simulink model "Microgrid_24h_Simulation"  (Simulink 9.3)
settings: Solver=ode45  StartTime=0.0  StopTime=1  RelTol=1e-3  EnableMultiTasking=on
undefined symbols (not defined in the file or in its folder): Acid, Lead
libraries: powerlib x60, powerlib_extras x56, simulink x3, powerlib_meascontrol x2, electricdrivelib x1
(part 1 of 3)
settings Model: Creator=Student  LastModifiedBy=DELL
settings DataIOCC: LimitDataPoints=on
settings OptimizationCC: ExpressionDepthLimit=2147483647
settings DebuggingCC: SolverPrmCheckMsg=warning  StateNameClashWarn=warning
settings GRTTargetCC: GeneratePreprocessorConditionals=Disable all
settings SimscapeCC: SimscapeNormalizeSystem=off

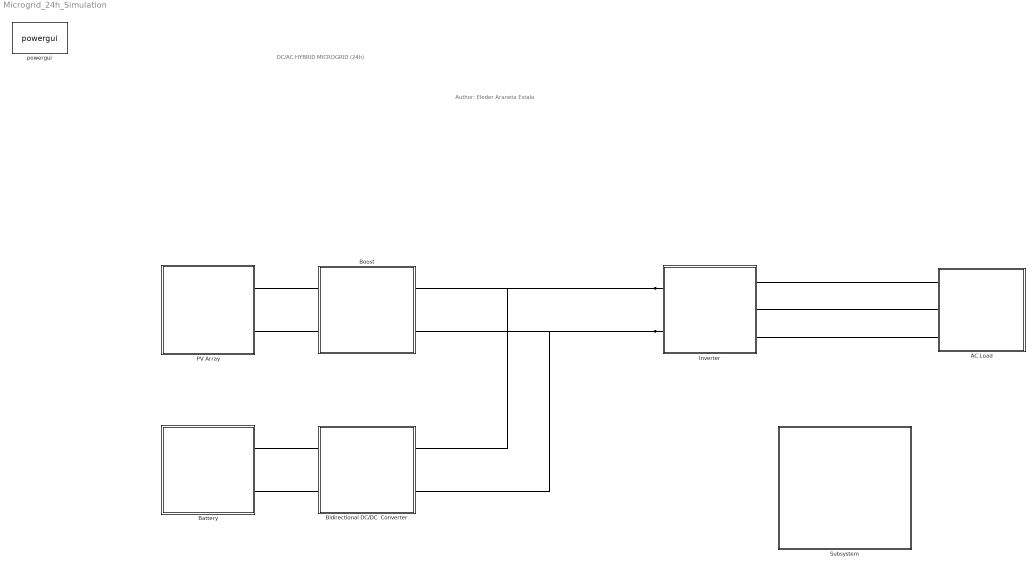
== system Microgrid_24h_Simulation ==
  note: DC/AC HYBRID MICROGRID (24h)
  note: Author: Eleder Araneta Estala
  AC Load : Subsystem
      mask Display: image(imread('Plug.bmp'))
  Battery : Subsystem
      mask Display: image(imread('Battery.bmp'))
  Bidirectional DC/DC  Converter : Subsystem
      mask Display: disp('Bidirectional Converter')
  Boost : Subsystem
      mask Display: disp('Boost Converter')
  Inverter : Subsystem
      mask Display: disp('DC/AC Inverter')
  PV Array : Subsystem
      mask Display: image(imread('photo.bmp'))
  Subsystem : Subsystem
      mask Display: disp('Measurements')
  powergui : powerlib/powergui  Priority=1  SimulationMode=Discrete  SampleTime=5e-6  frequency=60  Iterations=50  frequencyindice=0  Pbase=100e6  ErrMax=1e-4  UnitsV=kV  UnitsW=MW  buscounter=0  FunctionMessages=off  echomessages=off  EnableUseOfTLC=off  CurrentSourceSwitches=off  DisableSnubberDevices=off  DisableRonSwitches=off  DisableVfSwitches=off  DisplayEquations=off  AutomaticDiscreteSolvers=off  SolverType=Tustin  Interpol=off  ExternalGateDelay=off  methode=off  Ts=0  x0status=blocks  SPID=off  SwTol=0  HookPort=off  NonlinearTolerance=0  nMaxIteration=15  ContinueOnMaxIteration=off  RestoreLinks=warning  ResistiveCurrentMeasurement=off  Frange=[0:2:500]  Ylog=off  Xlog=on  ShowGrid=off  save=off  variable=ZData  structure=Vab_st  ZoomFFT=off  StartTime=7.5  cycles=4  DisplayStyle=1  fundamental=50  FreqAxis=off  MaxFrequency=50000  frequencyindicesteady=1  RmsSteady=1  display=off
      settings: SourceProductName=Simscape Electrical
  connections:
  Battery/LConn1 -- Bidirectional DC/DC  Converter/LConn1
  Battery/LConn2 -- Bidirectional DC/DC  Converter/LConn2
  PV Array/RConn2 -- Boost/LConn2
  PV Array/RConn1 -- Boost/LConn1
  Inverter/RConn1 -- Boost/RConn1 -- Bidirectional DC/DC  Converter/RConn1
  Inverter/RConn2 -- Boost/RConn2 -- Bidirectional DC/DC  Converter/RConn2
  AC Load/LConn3 -- Inverter/LConn3
  AC Load/LConn2 -- Inverter/LConn2
  AC Load/LConn1 -- Inverter/LConn1

== system Microgrid_24h_Simulation/AC Load ==
  3-Phase Dynamic Load : powerlib/Elements/Three-Phase Dynamic Load  NominalVoltage=[ 400 50 ]  ActiveReactivePowers=[25000 -500]  PositiveSequence=[1 0]  ExternalControl=off  NpNq="[1  1]"  TimeConstants="[0  0  0  0]"  MinimumVoltage=0.7  Tfilter=1e-4  LoadFlowParameters=[4 50000000 0 0 25000000]
      settings: SourceProductName=Simscape Electrical  SourceProductBaseCode=PS
  Bus Selector1 : BusSelector  OutputSignals=Active power P (W),Reactive power Q (var)  OutputAsBus=on
  Load Measurements : Subsystem
  Load Measurements1 : Subsystem
  Load Measurements2 : Scope
  Three-Phase Parallel RLC Load1 : powerlib/Elements/Three-Phase Parallel RLC Load  LConnTagsString=A|B|C  Configuration=Y (grounded)  NominalVoltage=400  Vabc=[1e3 1e3 1e3]  Vabcp=[1e3 1e3 1e3]  NominalFrequency=50  UnbalancedPower=off  ActivePower=700e3  InductivePower=0  CapacitivePower=0  Pabc=[10e3 9e3 11e3]  QLabc=[100 90 110]  QCabc=[100 90 110]  Pabcp=[10e3 9e3 11e3]  QLabcp=[100 90 110]  QCabcp=[100 90 110]  Measurements=Branch voltages and currents  LoadType=constant Z
      settings: SourceProductName=Simscape Electrical
  A : PMIOPort  Side=Left
  B : PMIOPort  Port=2  Side=Left
  C : PMIOPort  Port=3  Side=Left
  wires:
  3-Phase Dynamic Load/1 -> Bus Selector1/1
  Bus Selector1/1 -> Load Measurements2/1
  connections:
  A/RConn1 -- Load Measurements/LConn1 -- Load Measurements1/LConn1
  Load Measurements/LConn2 -- B/RConn1 -- Load Measurements1/LConn2
  Load Measurements/LConn3 -- C/RConn1 -- Load Measurements1/LConn3
  Load Measurements1/RConn1 -- Three-Phase Parallel RLC Load1/LConn1
  Load Measurements1/RConn2 -- Three-Phase Parallel RLC Load1/LConn2
  Load Measurements1/RConn3 -- Three-Phase Parallel RLC Load1/LConn3
  Load Measurements/RConn1 -- 3-Phase Dynamic Load/LConn1
  Load Measurements/RConn2 -- 3-Phase Dynamic Load/LConn2
  Load Measurements/RConn3 -- 3-Phase Dynamic Load/LConn3

== system Microgrid_24h_Simulation/Battery ==
  Battery : electricdrivelib/Extra Sources/Battery  BatType=Lead-Acid  ShowTempParam=off  ThermalPreset=no  ShowAgeParam=off  NomV=250  NomQ=500  SOC=30  Batt_Tr=1  PresetModel=on  MaxQ=520.8333  MinV=187.5  FullV=272.2039  Dis_rate=100  R=0.005  Normal_OP=155.1389  expZone="[254.523      1.666667]"  current=[20 50 100]  Units=Time  Tci=20  NomT=20  T2=-30  MaxQ2=4.8  FullV2=7.1  Normal_OP2=5.655  expZone2="[6.58           1]"  Rca=0.6  ti=2000  Dp=0  Neq0=0  Tsim=1e6  Ta1=25  Qeol=5.4*0.9  Reol=0.013333*1.2  Char_age=[2.3478, 3]  Dis_age=[2.3478, 10]  N1=1500  N2=10500  N3=1000  N4=1400  Ta2=45  N5=950
      settings: SourceProductName=Simscape Electrical
  Bus Selector : BusSelector  OutputSignals=SOC (%),Current (A),Voltage (V)
  LPF vq1 : powerlib_extras/Discrete  Control Blocks/Discrete 1st-Order Filter  FilterType=Lowpass  Tc=10e-3  Ts=5e-6  Initialize=off  Vac_Init=[0.8 -25 60]  Vdc_Init=0  PlotResponse=off  param1=[1 100 0.1]
      settings: SourceProductName=Simscape Electrical  SourceProductBaseCode=PS
  LPF vq2 : powerlib_extras/Discrete  Control Blocks/Discrete 1st-Order Filter  FilterType=Lowpass  Tc=10e-3  Ts=5e-6  Initialize=off  Vac_Init=[0.8 -25 60]  Vdc_Init=0  PlotResponse=off  param1=[1 100 0.1]
      settings: SourceProductName=Simscape Electrical  SourceProductBaseCode=PS
  Subsystem1 : Subsystem
  Subsystem2 : Subsystem
  Subsystem5 : Subsystem
  + : PMIOPort  Side=Left
  - : PMIOPort  Port=2  Side=Left
  wires:
  Battery/1 -> Bus Selector/1
  Bus Selector/2 -> LPF vq1/1  "<Current (A)>"
  LPF vq1/1 -> Subsystem1/1(Ibat)
  Bus Selector/1 -> Subsystem5/1(SOC)  "<SOC (%)>"
  Bus Selector/3 -> LPF vq2/1  "<Voltage (V)>"
  LPF vq2/1 -> Subsystem2/1(Vbat)
  connections:
  -/RConn1 -- Battery/LConn2
  Battery/LConn1 -- +/RConn1

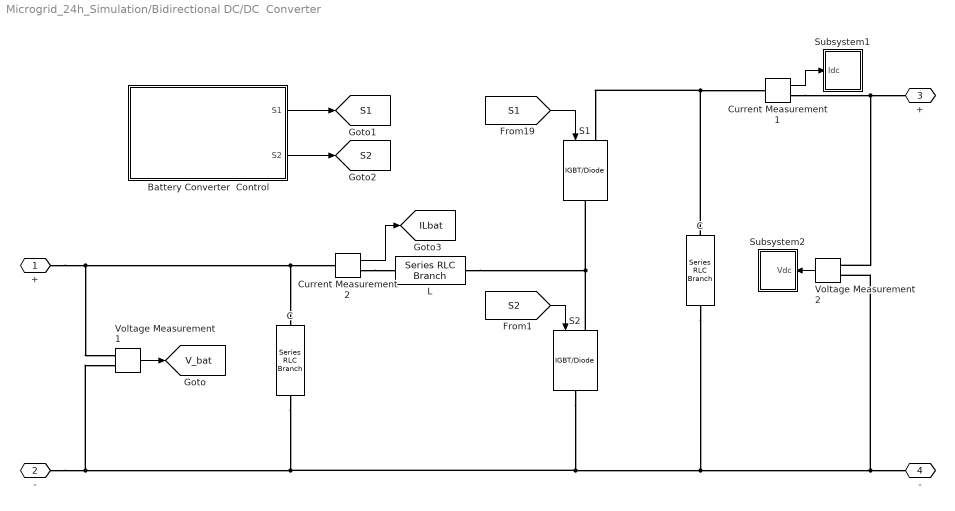
== system Microgrid_24h_Simulation/Bidirectional DC/DC  Converter ==
  Battery Converter  Control : Subsystem
  C : powerlib/Elements/Series RLC Branch  LConnTagsString=__new0  RConnTagsString=__new0  BranchType=C  Resistance=1  Inductance=1e-3  SetiL0=off  InitialCurrent=0  Capacitance=1200e-6  Setx0=off  InitialVoltage=400  Measurements=None
      settings: SourceProductName=Simscape Electrical
  "C " : powerlib/Elements/Series RLC Branch  LConnTagsString=__new0  RConnTagsString=__new0  BranchType=C  Resistance=1  Inductance=1e-3  SetiL0=off  InitialCurrent=0  Capacitance=1e-3  Setx0=on  InitialVoltage=192  Measurements=None
      settings: SourceProductName=Simscape Electrical
  Current Measurement1 : powerlib/Measurements/Current Measurement  PhasorSimulation=off  OutputType=Complex  PSBequivalent=0
      settings: SourceProductName=Simscape Electrical
  Current Measurement2 : powerlib/Measurements/Current Measurement  PhasorSimulation=off  OutputType=Complex  PSBequivalent=0
      settings: SourceProductName=Simscape Electrical
  L : powerlib/Elements/Series RLC Branch  LConnTagsString=__new0  RConnTagsString=__new0  BranchType=L  Resistance=1  Inductance=0.1e-3  SetiL0=on  InitialCurrent=0  Capacitance=1e-6  Setx0=off  InitialVoltage=0  Measurements=None
      settings: SourceProductName=Simscape Electrical
  "S1 " : powerlib/Power Electronics/IGBT//Diode  Ron=1e-3  Rs=1e5  Cs=inf  Measurements=off
      settings: SourceProductName=Simscape Electrical
  "S2 " : powerlib/Power Electronics/IGBT//Diode  Ron=1e-3  Rs=1e5  Cs=inf  Measurements=off
      settings: SourceProductName=Simscape Electrical
  Subsystem1 : Subsystem
  Subsystem2 : Subsystem
  Voltage Measurement1 : powerlib/Measurements/Voltage Measurement  PhasorSimulation=off  OutputType=Complex  PSBequivalent=0
      settings: SourceProductName=Simscape Electrical
  Voltage Measurement2 : powerlib/Measurements/Voltage Measurement  PhasorSimulation=off  OutputType=Complex  PSBequivalent=0
      settings: SourceProductName=Simscape Electrical
  "+ " : PMIOPort  Side=Left
  "-  " : PMIOPort  Port=2  Side=Left
  + : PMIOPort  Port=3  Side=Right
  - : PMIOPort  Port=4  Side=Right
  tag scope: ILbat=global, S1=global, S2=global, V_bat=global
  wires:
  Voltage Measurement1/1 -> [V_bat]
  Current Measurement2/1 -> [ILbat]
  Battery Converter  Control/1(S1) -> [S1]
  Battery Converter  Control/2(S2) -> [S2]
  [S1] -> "S1 "/1
  [S2] -> "S2 "/1
  Voltage Measurement2/1 -> Subsystem2/1(Vdc)
  Current Measurement1/1 -> Subsystem1/1(Idc)
  connections:
  "-  "/RConn1 -- Voltage Measurement1/LConn2 -- "C "/RConn1 -- "S2 "/RConn1 -- C/RConn1 -- -/RConn1 -- Voltage Measurement2/LConn2
  "S2 "/LConn1 -- "S1 "/RConn1 -- L/RConn1
  C/LConn1 -- "S1 "/LConn1 -- Current Measurement1/LConn1
  Current Measurement2/RConn1 -- L/LConn1
  "+ "/RConn1 -- Voltage Measurement1/LConn1 -- Current Measurement2/LConn1 -- "C "/LConn1
  Current Measurement1/RConn1 -- +/RConn1 -- Voltage Measurement2/LConn1

== system Microgrid_24h_Simulation/Boost ==
  Cdc : powerlib/Elements/Series RLC Branch  LConnTagsString=__new0  RConnTagsString=__new0  BranchType=C  Resistance=1  Inductance=1e-3  SetiL0=off  InitialCurrent=0  Capacitance=1200e-6  Setx0=off  InitialVoltage=400  Measurements=None
      settings: SourceProductName=Simscape Electrical
  Current Measurement : powerlib/Measurements/Current Measurement  PhasorSimulation=off  OutputType=Complex  PSBequivalent=0
      settings: SourceProductName=Simscape Electrical
  Current Measurement1 : powerlib/Measurements/Current Measurement  PhasorSimulation=off  OutputType=Complex  PSBequivalent=0
      settings: SourceProductName=Simscape Electrical
  Diode : powerlib/Power Electronics/Diode  Ron=0.001  Lon=0  Vf=0.8  IC=0  UseSnubber=off  Rs=500  Cs=250e-9  Measurements=on
      settings: SourceProductName=Simscape Electrical
  IGBT/Diode : powerlib/Power Electronics/IGBT//Diode  Ron=1e-3  Rs=1e5  Cs=inf  Measurements=off
      settings: SourceProductName=Simscape Electrical
  Incremental Conductance MPPT : Subsystem
  Lb : powerlib/Elements/Series RLC Branch  LConnTagsString=__new0  RConnTagsString=__new0  BranchType=L  Resistance=1  Inductance=880e-6  SetiL0=off  InitialCurrent=0  Capacitance=1e-6  Setx0=off  InitialVoltage=0  Measurements=None
      settings: SourceProductName=Simscape Electrical
  Subsystem1 : Subsystem
  Subsystem2 : Subsystem
  Va : powerlib/Measurements/Voltage Measurement  PhasorSimulation=off  OutputType=Complex  PSBequivalent=0
      settings: SourceProductName=Simscape Electrical
  Voltage Measurement : powerlib/Measurements/Voltage Measurement  PhasorSimulation=off  OutputType=Complex  PSBequivalent=0
      settings: SourceProductName=Simscape Electrical
  + : PMIOPort  Side=Left
  - : PMIOPort  Port=2  Side=Left
  "+ " : PMIOPort  Port=3  Side=Right
  "- " : PMIOPort  Port=4  Side=Right
  tag scope: IL=global, S=global, Vin=global
  wires:
  Current Measurement/1 -> [IL]
  [S] -> IGBT/Diode/1
  Voltage Measurement/1 -> Subsystem2/1(Vbus)
  Current Measurement1/1 -> Subsystem1/1(Ibus)
  Va/1 -> [Vin]
  Incremental Conductance MPPT/1(Pulsos) -> [S]
  connections:
  Voltage Measurement/LConn1 -- Current Measurement1/LConn1 -- Diode/RConn1 -- Cdc/LConn1
  Cdc/RConn1 -- "- "/RConn1 -- Voltage Measurement/LConn2 -- -/RConn1 -- Va/LConn2 -- IGBT/Diode/RConn1
  Lb/RConn1 -- Current Measurement/LConn1
  IGBT/Diode/LConn1 -- Current Measurement/RConn1 -- Diode/LConn1
  +/RConn1 -- Lb/LConn1 -- Va/LConn1
  "+ "/RConn1 -- Current Measurement1/RConn1

== system Microgrid_24h_Simulation/Inverter ==
  DC / AC Inverter : Subsystem
  "DC BUS " : Subsystem
  Inverter Control : Subsystem
  Inverter Control1 : Subsystem
  + : PMIOPort  Side=Right
  A : PMIOPort  Port=2  Side=Left
  B : PMIOPort  Port=3  Side=Left
  - : PMIOPort  Port=4  Side=Right
  C : PMIOPort  Port=5  Side=Left
  wires:
  Inverter Control/1(S) -> DC / AC Inverter/1(S)
  connections:
  A/RConn1 -- DC / AC Inverter/LConn1
  B/RConn1 -- DC / AC Inverter/LConn2
  C/RConn1 -- DC / AC Inverter/LConn3
  "DC BUS "/LConn2 -- DC / AC Inverter/RConn2
  "DC BUS "/LConn1 -- DC / AC Inverter/RConn1
  +/RConn1 -- "DC BUS "/RConn1
  -/RConn1 -- "DC BUS "/RConn2

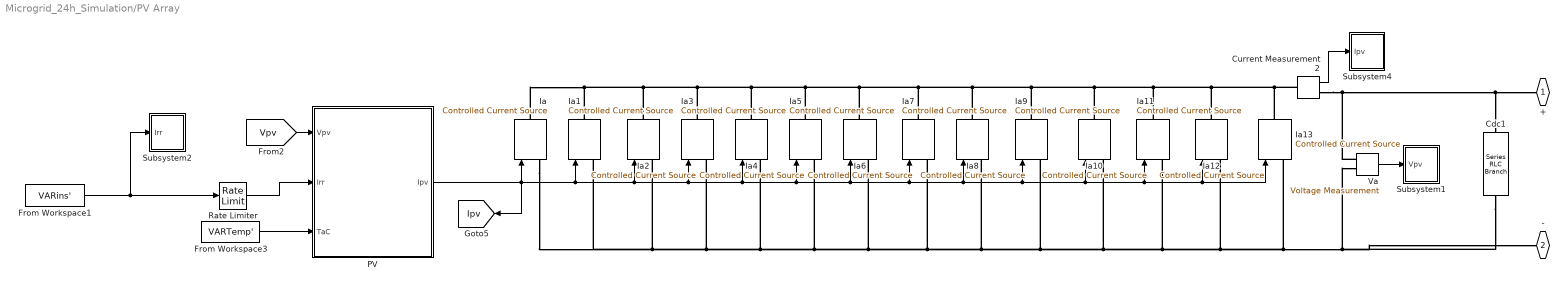
== system Microgrid_24h_Simulation/PV Array ==
  Cdc1 : powerlib/Elements/Series RLC Branch  LConnTagsString=__new0  RConnTagsString=__new0  BranchType=C  Resistance=1  Inductance=1e-3  SetiL0=off  InitialCurrent=0  Capacitance=5e-3  Setx0=off  InitialVoltage=192  Measurements=None
      settings: SourceProductName=Simscape Electrical
  Current Measurement2 : powerlib/Measurements/Current Measurement  PhasorSimulation=off  OutputType=Complex  PSBequivalent=0
      settings: SourceProductName=Simscape Electrical
  From Workspace1 : FromWorkspace  VariableName=VARins'  SampleTime=0
  From Workspace3 : FromWorkspace  VariableName=VARTemp'  SampleTime=0
  Ia{,1..13} (14 alike) : powerlib/Electrical Sources/Controlled Current Source  Initialize=on  Source_Type=DC  Amplitude=0  Phase=0  Frequency=0  Measurements=None
      settings: SourceProductName=Simscape Electrical
  PV : MATLAB Function  TreatAsAtomicUnit=on
  Rate Limiter : RateLimiter  RisingSlewLimit=5  FallingSlewLimit=-5
  Subsystem1 : Subsystem
  Subsystem2 : Subsystem
  Subsystem4 : Subsystem
  Va : powerlib/Measurements/Voltage Measurement  PhasorSimulation=off  OutputType=Complex  PSBequivalent=0
      settings: SourceProductName=Simscape Electrical
  + : PMIOPort  Side=Right
  - : PMIOPort  Port=2  Side=Right
  tag scope: Ipv=global
  wires:
  [Vpv] -> PV/1(Vpv)
  PV/1(Ipv) -> Ia/1, [Ipv], Ia1/1, Ia2/1, Ia3/1, Ia4/1, Ia5/1, Ia6/1, Ia7/1, Ia8/1, Ia9/1, Ia10/1, Ia11/1, Ia13/1, Ia12/1
  Va/1 -> Subsystem1/1(Vpv)
  Rate Limiter/1 -> PV/2(Irr)
  Current Measurement2/1 -> Subsystem4/1(Ipv)
  From Workspace3/1 -> PV/3(TaC)
  From Workspace1/1 -> Subsystem2/1(Irr), Rate Limiter/1
  connections:
  Ia/LConn1 -- Ia1/LConn1 -- Ia2/LConn1 -- Ia3/LConn1 -- Ia4/LConn1 -- Ia5/LConn1 -- Ia6/LConn1 -- Ia7/LConn1 -- Ia8/LConn1 -- Ia9/LConn1 -- Ia10/LConn1 -- Ia11/LConn1 -- Ia12/LConn1 -- Va/LConn2 -- Cdc1/RConn1 -- -/RConn1 -- Ia13/LConn1
  Current Measurement2/LConn1 -- Ia/RConn1 -- Ia1/RConn1 -- Ia2/RConn1 -- Ia3/RConn1 -- Ia4/RConn1 -- Ia5/RConn1 -- Ia6/RConn1 -- Ia7/RConn1 -- Ia8/RConn1 -- Ia9/RConn1 -- Ia10/RConn1 -- Ia11/RConn1 -- Ia12/RConn1 -- Ia13/RConn1
  Va/LConn1 -- Current Measurement2/RConn1 -- +/RConn1 -- Cdc1/LConn1

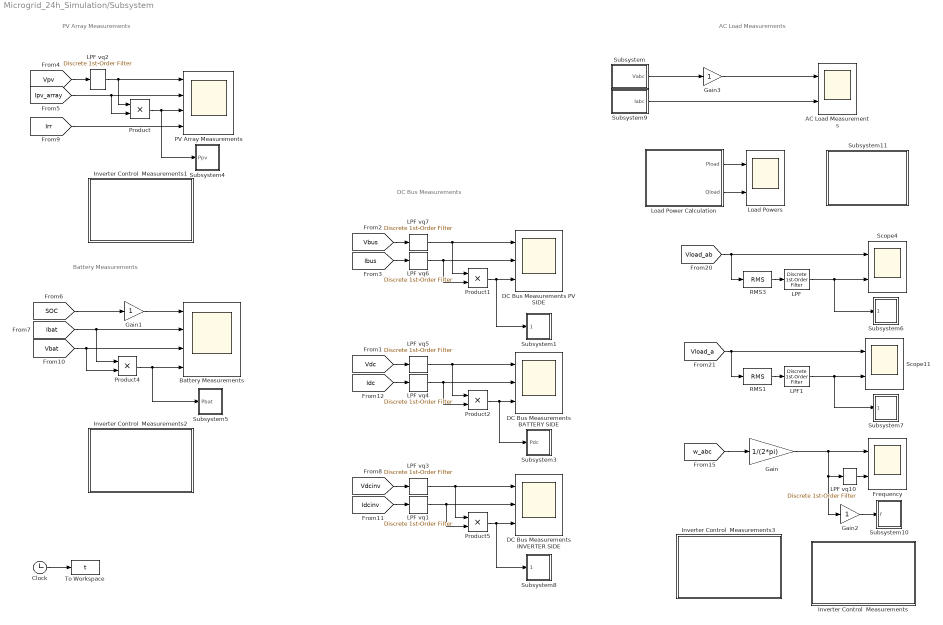
== system Microgrid_24h_Simulation/Subsystem ==
  note: PV Array Measurements
  note: Battery Measurements
  note: DC Bus Measurements
  note: AC Load Measurements
  AC Load Measurements : Scope  NumInputPorts=2
  Battery Measurements : Scope  NumInputPorts=4
  Clock : Clock
  DC Bus Measurements BATTERY SIDE : Scope  NumInputPorts=3
  DC Bus Measurements INVERTER SIDE : Scope  NumInputPorts=3
  DC Bus Measurements PV SIDE : Scope  NumInputPorts=3
  Frequency : Scope  NumInputPorts=2
  Gain : Gain  Gain=1/(2*pi)
  Gain1 : Gain
  Gain2 : Gain
  Gain3 : Gain
  Inverter Control  Measurements : Subsystem
      mask Display: disp('Inverter Control')
  Inverter Control  Measurements1 : Subsystem
      mask Display: disp('Boost Converter Control')
  Inverter Control  Measurements2 : Subsystem
      mask Display: disp('Bidirectional Converter Control')
  Inverter Control  Measurements3 : Subsystem
      mask Display: disp('Frequency Measurement')
  LPF : powerlib_extras/Discrete  Control Blocks/Discrete 1st-Order Filter  FilterType=Lowpass  Tc=10e-3  Ts=5e-6  Initialize=off  Vac_Init=[0.8 -25 60]  Vdc_Init=0  PlotResponse=off  param1=[1 100 0.1]
      settings: SourceProductName=Simscape Electrical  SourceProductBaseCode=PS
  LPF vq{1..7,10} (8 alike) : powerlib_extras/Discrete  Control Blocks/Discrete 1st-Order Filter  FilterType=Lowpass  Tc=10e-3  Ts=5e-6  Initialize=off  Vac_Init=[0.8 -25 60]  Vdc_Init=0  PlotResponse=off  param1=[1 100 0.1]
      settings: SourceProductName=Simscape Electrical  SourceProductBaseCode=PS
  LPF1 : powerlib_extras/Discrete  Control Blocks/Discrete 1st-Order Filter  FilterType=Lowpass  Tc=10e-3  Ts=5e-6  Initialize=off  Vac_Init=[0.8 -25 60]  Vdc_Init=0  PlotResponse=off  param1=[1 100 0.1]
      settings: SourceProductName=Simscape Electrical  SourceProductBaseCode=PS
  Load Power Calculation : Subsystem
  Load Powers : Scope  NumInputPorts=2
  PV Array Measurements : Scope  NumInputPorts=4
  Product{,1..2,4..5} (5 alike) : Product  RndMeth=Zero
  RMS1 : powerlib_extras/Measurements/RMS  f1=60
      settings: SourceProductName=Simscape Electrical  SourceProductBaseCode=PS
  RMS3 : powerlib_extras/Measurements/RMS  f1=60
      settings: SourceProductName=Simscape Electrical  SourceProductBaseCode=PS
  Scope11 : Scope  NumInputPorts=2
  Scope4 : Scope  NumInputPorts=2
  Subsystem : Subsystem
  Subsystem1 : Subsystem
  Subsystem10 : Subsystem
  Subsystem11 : Subsystem
      mask Display: disp('Additional Load Meas.')
  Subsystem3 : Subsystem
  Subsystem4 : Subsystem
  Subsystem5 : Subsystem
  Subsystem6 : Subsystem
  Subsystem7 : Subsystem
  Subsystem8 : Subsystem
  Subsystem9 : Subsystem
  To Workspace : ToWorkspace  VariableName=t  SampleTime=5e-6
  wires:
  Product/1 -> PV Array Measurements/3, Subsystem4/1(Ppv)
  [Vpv] -> LPF vq2/1
  [Ipv_array] -> PV Array Measurements/2, Product/2
  [Irr] -> PV Array Measurements/4
  [SOC] -> Gain1/1
  [Ibat] -> Battery Measurements/2, Product4/1
  [Vbat] -> Battery Measurements/3, Product4/2
  Product4/1 -> Battery Measurements/4, Subsystem5/1(Pbat)
  [Vdc] -> LPF vq5/1
  [Idc] -> LPF vq4/1
  Product2/1 -> DC Bus Measurements BATTERY SIDE/3, Subsystem3/1(Pdc)
  Product1/1 -> DC Bus Measurements PV SIDE/3, Subsystem1/1(Pbus)
  [Vbus] -> LPF vq7/1
  [Ibus] -> LPF vq6/1
  Load Power Calculation/1(Pload) -> Load Powers/1
  Load Power Calculation/2(Qload) -> Load Powers/2
  [Vload_a] -> Scope11/1, RMS1/1
  RMS1/1 -> LPF1/1
  [Vload_ab] -> Scope4/1, RMS3/1
  RMS3/1 -> LPF/1
  LPF/1 -> Scope4/2, Subsystem6/1(Vab_rms)
  LPF1/1 -> Scope11/2, Subsystem7/1(Va_rms)
  Clock/1 -> To Workspace/1
  Product5/1 -> Subsystem8/1(Pdcinv), DC Bus Measurements INVERTER SIDE/3
  [Vdcinv] -> LPF vq3/1
  [Idcinv] -> LPF vq1/1
  LPF vq2/1 -> PV Array Measurements/1, Product/1
  LPF vq1/1 -> DC Bus Measurements INVERTER SIDE/2, Product5/2
  LPF vq3/1 -> DC Bus Measurements INVERTER SIDE/1, Product5/1
  LPF vq4/1 -> Product2/2, DC Bus Measurements BATTERY SIDE/2
  LPF vq5/1 -> Product2/1, DC Bus Measurements BATTERY SIDE/1
  LPF vq6/1 -> DC Bus Measurements PV SIDE/2, Product1/2
  LPF vq7/1 -> DC Bus Measurements PV SIDE/1, Product1/1
  [w_abc] -> Gain/1
  Gain/1 -> Frequency/1, LPF vq10/1, Gain2/1
  LPF vq10/1 -> Frequency/2
  Subsystem9/1(Iabc) -> AC Load Measurements/2
  Subsystem/1(Vabc) -> Gain3/1
  Gain1/1 -> Battery Measurements/1
  Gain2/1 -> Subsystem10/1(f)
  Gain3/1 -> AC Load Measurements/1

== system Microgrid_24h_Simulation/AC Load/Load Measurements ==
  Subsystem1 : Subsystem
  Subsystem2 : Subsystem
  Three-Phase V Measurement : powerlib/Measurements/Three-Phase V-I Measurement  VoltageMeasurement=phase-to-ground  SetLabelV=off  LabelV=Vabc  Vpu=off  VpuLL=off  CurrentMeasurement=no  SetLabelI=off  LabelI=Iabc  Ipu=off  Pbase=100e6  Vbase=500e3  OutputType=Complex  PhasorSimulation=off  PSBequivalent=0
      settings: SourceProductName=Simscape Electrical
  Three-Phase  I Measurement : powerlib/Measurements/Three-Phase V-I Measurement  VoltageMeasurement=no  SetLabelV=off  LabelV=Vabc  Vpu=off  VpuLL=off  CurrentMeasurement=yes  SetLabelI=off  LabelI=Iabc  Ipu=off  Pbase=100e6  Vbase=500e3  OutputType=Complex  PhasorSimulation=off  PSBequivalent=0
      settings: SourceProductName=Simscape Electrical
  A : PMIOPort  Side=Left
  "A " : PMIOPort  Port=2  Side=Right
  B : PMIOPort  Port=3  Side=Left
  "B " : PMIOPort  Port=4  Side=Right
  C : PMIOPort  Port=5  Side=Left
  "C " : PMIOPort  Port=6  Side=Right
  wires:
  Three-Phase  I Measurement/1 -> Subsystem2/1(Iabc)
  Three-Phase V Measurement/1 -> Subsystem1/1(Vabc)
  connections:
  Three-Phase V Measurement/LConn1 -- Three-Phase  I Measurement/RConn1
  Three-Phase V Measurement/LConn2 -- Three-Phase  I Measurement/RConn2
  Three-Phase  I Measurement/RConn3 -- Three-Phase V Measurement/LConn3
  A/RConn1 -- Three-Phase  I Measurement/LConn1
  Three-Phase V Measurement/RConn1 -- "A "/RConn1
  B/RConn1 -- Three-Phase  I Measurement/LConn2
  Three-Phase V Measurement/RConn2 -- "B "/RConn1
  C/RConn1 -- Three-Phase  I Measurement/LConn3
  Three-Phase V Measurement/RConn3 -- "C "/RConn1

== system Microgrid_24h_Simulation/AC Load/Load Measurements1 ==
  Subsystem1 : Subsystem
  Subsystem2 : Subsystem
  Three-Phase V Measurement : powerlib/Measurements/Three-Phase V-I Measurement  VoltageMeasurement=phase-to-ground  SetLabelV=off  LabelV=Vabc  Vpu=off  VpuLL=off  CurrentMeasurement=no  SetLabelI=off  LabelI=Iabc  Ipu=off  Pbase=100e6  Vbase=500e3  OutputType=Complex  PhasorSimulation=off  PSBequivalent=0
      settings: SourceProductName=Simscape Electrical
  Three-Phase  I Measurement : powerlib/Measurements/Three-Phase V-I Measurement  VoltageMeasurement=no  SetLabelV=off  LabelV=Vabc  Vpu=off  VpuLL=off  CurrentMeasurement=yes  SetLabelI=off  LabelI=Iabc  Ipu=off  Pbase=100e6  Vbase=500e3  OutputType=Complex  PhasorSimulation=off  PSBequivalent=0
      settings: SourceProductName=Simscape Electrical
  a : PMIOPort  Side=Left
  "A " : PMIOPort  Port=2  Side=Right
  B : PMIOPort  Port=3  Side=Left
  "B " : PMIOPort  Port=4  Side=Right
  C : PMIOPort  Port=5  Side=Left
  "C " : PMIOPort  Port=6  Side=Right
  wires:
  Three-Phase V Measurement/1 -> Subsystem1/1(Vabc)
  Three-Phase  I Measurement/1 -> Subsystem2/1(Iabc3)
  connections:
  Three-Phase V Measurement/RConn3 -- "C "/RConn1
  C/RConn1 -- Three-Phase  I Measurement/LConn3
  Three-Phase V Measurement/RConn2 -- "B "/RConn1
  B/RConn1 -- Three-Phase  I Measurement/LConn2
  Three-Phase V Measurement/RConn1 -- "A "/RConn1
  a/RConn1 -- Three-Phase  I Measurement/LConn1
  Three-Phase  I Measurement/RConn3 -- Three-Phase V Measurement/LConn3
  Three-Phase V Measurement/LConn2 -- Three-Phase  I Measurement/RConn2
  Three-Phase V Measurement/LConn1 -- Three-Phase  I Measurement/RConn1

== system Microgrid_24h_Simulation/Battery/Subsystem1 ==
  Ibat : Inport
  To Workspace1 : ToWorkspace  VariableName=Ibat  SampleTime=-1
  tag scope: Ibat=global
  wires:
  Ibat/1 -> To Workspace1/1, [Ibat]

== system Microgrid_24h_Simulation/Battery/Subsystem2 ==
  Vbat : Inport
  To Workspace1 : ToWorkspace  VariableName=Vbat  SampleTime=-1
  tag scope: Vbat=global
  wires:
  Vbat/1 -> To Workspace1/1, [Vbat]

== system Microgrid_24h_Simulation/Battery/Subsystem5 ==
  SOC : Inport
  To Workspace1 : ToWorkspace  VariableName=SOC  SampleTime=-1
  tag scope: SOC=global
  wires:
  SOC/1 -> To Workspace1/1, [SOC]

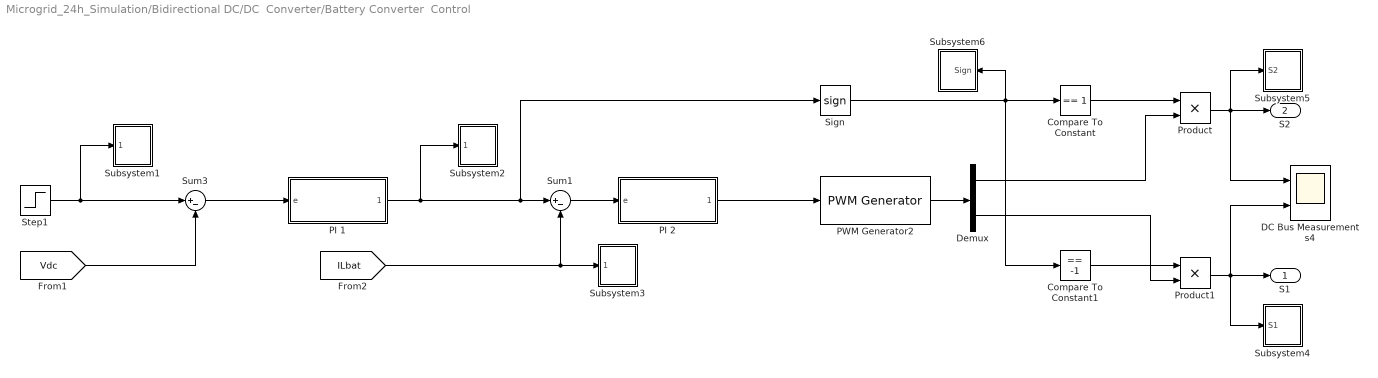
== system Microgrid_24h_Simulation/Bidirectional DC/DC  Converter/Battery Converter  Control ==
  Compare To Constant : simulink/Logic and Bit Operations/Compare To Constant  relop===  const=1  OutDataTypeStr=uint8
  Compare To Constant1 : simulink/Logic and Bit Operations/Compare To Constant  relop===  const=-1  OutDataTypeStr=uint8
  DC Bus Measurements4 : Scope  NumInputPorts=2
  Demux : Demux  Outputs=2
  PI 1 : Subsystem
  PI 2 : Subsystem
  PWM Generator2 : powerlib_extras/Control  Blocks/PWM Generator  GeneratorMode="1-arm  bridge (2 pulses)"  Fc=10000  Internal=off  mIndex=0.2  Freq=0  Phase=0
      link override Triangle: rep_seq_y=[0 1 0]  rep_seq_t=[0 1/Fc/2 1/Fc]
      settings: SourceProductName=Simscape Electrical  SourceProductBaseCode=PS
  Product : Product  RndMeth=Zero
  Product1 : Product  RndMeth=Zero
  Sign : Signum  SampleTime=5e-6
  Step1 : Step  Time=0  After=1000  SampleTime=0
  Subsystem1 : Subsystem
  Subsystem2 : Subsystem
  Subsystem3 : Subsystem
  Subsystem4 : Subsystem
  Subsystem5 : Subsystem
  Subsystem6 : Subsystem
  Sum1 : Sum  Inputs=|+-
  Sum3 : Sum  Inputs=|+-
  S1 : Outport
  S2 : Outport  Port=2
  wires:
  Step1/1 -> Sum3/1, Subsystem1/1(Vdc_ref)
  Sum3/1 -> PI 1/1(e)
  Sum1/1 -> PI 2/1(e)
  [ILbat] -> Sum1/2, Subsystem3/1(ILbat)
  PI 1/1(" ") -> Sum1/1, Sign/1, Subsystem2/1(Ibat_ref)
  PI 2/1(" ") -> PWM Generator2/1
  PWM Generator2/1 -> Demux/1
  Sign/1 -> Compare To Constant/1, Compare To Constant1/1, Subsystem6/1(Sign)
  Compare To Constant/1 -> Product/1
  Demux/1 -> Product/2
  Compare To Constant1/1 -> Product1/1
  Product/1 -> DC Bus Measurements4/1, S2/1, Subsystem5/1(S2)
  Product1/1 -> S1/1, Subsystem4/1(S1), DC Bus Measurements4/2
  Demux/2 -> Product1/2
  [Vdc] -> Sum3/2

== system Microgrid_24h_Simulation/Bidirectional DC/DC  Converter/Subsystem1 ==
  Idc : Inport
  LPF vq11 : powerlib_extras/Discrete  Control Blocks/Discrete 1st-Order Filter  FilterType=Lowpass  Tc=10e-3  Ts=5e-6  Initialize=off  Vac_Init=[0.8 -25 60]  Vdc_Init=0  PlotResponse=off  param1=[1 100 0.1]
      settings: SourceProductName=Simscape Electrical  SourceProductBaseCode=PS
  To Workspace1 : ToWorkspace  VariableName=Idc  SampleTime=-1
  To Workspace2 : ToWorkspace  VariableName=Idc1  SampleTime=-1
  tag scope: Idc=global
  wires:
  Idc/1 -> [Idc], To Workspace1/1, LPF vq11/1
  LPF vq11/1 -> To Workspace2/1

== system Microgrid_24h_Simulation/Bidirectional DC/DC  Converter/Subsystem2 ==
  Vdc : Inport
  LPF vq11 : powerlib_extras/Discrete  Control Blocks/Discrete 1st-Order Filter  FilterType=Lowpass  Tc=10e-3  Ts=5e-6  Initialize=off  Vac_Init=[0.8 -25 60]  Vdc_Init=0  PlotResponse=off  param1=[1 100 0.1]
      settings: SourceProductName=Simscape Electrical  SourceProductBaseCode=PS
  To Workspace1 : ToWorkspace  VariableName=Vdc  SampleTime=-1
  To Workspace2 : ToWorkspace  VariableName=Vdc1  SampleTime=-1
  tag scope: Vdc=global
  wires:
  Vdc/1 -> [Vdc], To Workspace1/1, LPF vq11/1
  LPF vq11/1 -> To Workspace2/1

== system Microgrid_24h_Simulation/Boost/Incremental Conductance MPPT ==
  Demux : Demux  Outputs=2
  MPPT IC : MATLAB Function  TreatAsAtomicUnit=on
  Memory{,1..2,4..5} (5 alike) : Memory
  PWM Generator : powerlib_extras/Control  Blocks/PWM Generator  GeneratorMode="1-arm  bridge (2 pulses)"  Fc=10e3  Internal=off  mIndex=0.4  Freq=60  Phase=0
      link override Triangle: rep_seq_t=[0 1/Fc/2 1/Fc]  rep_seq_y=[0 1 0]
      settings: SourceProductName=Simscape Electrical  SourceProductBaseCode=PS
  Subsystem1 : Subsystem
  Subsystem2 : Subsystem
  Subsystem3 : Subsystem
  Pulsos : Outport
  wires:
  Memory2/1 -> MPPT IC/4(Vprevious)
  Memory5/1 -> MPPT IC/5(Vref_previous)
  Memory4/1 -> MPPT IC/2(Iprevious)
  Memory1/1 -> MPPT IC/3(Vpv)
  Memory/1 -> MPPT IC/1(Ipv)
  PWM Generator/1 -> Demux/1
  Demux/2 -> Pulsos/1, Subsystem3/1(pulsos)
  MPPT IC/1(delta) -> Subsystem2/1(delta), PWM Generator/1
  MPPT IC/3(Ipv_prev_out) -> Memory4/1
  MPPT IC/4(Vpv_prev_out) -> Memory2/1
  MPPT IC/2(Vref) -> Memory5/1, Subsystem1/1(Vref)
  [Ipv] -> Memory/1
  [Vpv] -> Memory1/1

== system Microgrid_24h_Simulation/Boost/Subsystem1 ==
  Ibus : Inport
  LPF vq11 : powerlib_extras/Discrete  Control Blocks/Discrete 1st-Order Filter  FilterType=Lowpass  Tc=10e-3  Ts=5e-6  Initialize=off  Vac_Init=[0.8 -25 60]  Vdc_Init=0  PlotResponse=off  param1=[1 100 0.1]
      settings: SourceProductName=Simscape Electrical  SourceProductBaseCode=PS
  To Workspace1 : ToWorkspace  VariableName=Ibus  SampleTime=-1
  To Workspace2 : ToWorkspace  VariableName=Ibus1  SampleTime=-1
  tag scope: Ibus=global
  wires:
  Ibus/1 -> [Ibus], To Workspace1/1, LPF vq11/1
  LPF vq11/1 -> To Workspace2/1

== system Microgrid_24h_Simulation/Boost/Subsystem2 ==
  Vbus : Inport
  LPF vq11 : powerlib_extras/Discrete  Control Blocks/Discrete 1st-Order Filter  FilterType=Lowpass  Tc=10e-3  Ts=5e-6  Initialize=off  Vac_Init=[0.8 -25 60]  Vdc_Init=0  PlotResponse=off  param1=[1 100 0.1]
      settings: SourceProductName=Simscape Electrical  SourceProductBaseCode=PS
  To Workspace1 : ToWorkspace  VariableName=Vbus  SampleTime=-1
  To Workspace2 : ToWorkspace  VariableName=Vbus1  SampleTime=-1
  tag scope: Vbus=global
  wires:
  Vbus/1 -> [Vbus], To Workspace1/1, LPF vq11/1
  LPF vq11/1 -> To Workspace2/1

== system Microgrid_24h_Simulation/Inverter/DC / AC Inverter ==
  S : Inport
  2 Level Inverter : powerlib/Power Electronics/Universal Bridge  Arms=3  SnubberResistance=1e5  SnubberCapacitance=inf  Device=IGBT / Diodes  Ron=1e-3  Lon=0  ForwardVoltages="[  0  0  ]"  ForwardVoltage=0  GTOparameters=[ 10e-6 , 20e-6 ]  IGBTparameters=[ 1e-6 , 2e-6 ]  Measurements=UAB UBC UCA UDC voltages  Measurements_2=None  converterType=Rectifier
      settings: SourceProductName=Simscape Electrical
  AC Load Measurements : Subsystem
  Series RLC Branch1 : powerlib/Elements/Series RLC Branch  LConnTagsString=__new0  RConnTagsString=__new0  BranchType=RL  Resistance=0.1  Inductance=30e-3  SetiL0=off  InitialCurrent=0  Capacitance=1e-6  Setx0=off  InitialVoltage=0  Measurements=Branch voltage
      settings: SourceProductName=Simscape Electrical
  Series RLC Branch2 : powerlib/Elements/Series RLC Branch  LConnTagsString=__new0  RConnTagsString=__new0  BranchType=RL  Resistance=0.1  Inductance=30e-3  SetiL0=off  InitialCurrent=0  Capacitance=1e-6  Setx0=off  InitialVoltage=0  Measurements=Branch voltage
      settings: SourceProductName=Simscape Electrical
  Series RLC Branch3 : powerlib/Elements/Series RLC Branch  LConnTagsString=__new0  RConnTagsString=__new0  BranchType=RL  Resistance=0.1  Inductance=30e-3  SetiL0=off  InitialCurrent=0  Capacitance=1e-6  Setx0=off  InitialVoltage=0  Measurements=Branch voltage
      settings: SourceProductName=Simscape Electrical
  + : PMIOPort  Side=Right
  A : PMIOPort  Port=2  Side=Left
  B : PMIOPort  Port=3  Side=Left
  - : PMIOPort  Port=4  Side=Right
  C : PMIOPort  Port=5  Side=Left
  wires:
  S/1 -> 2 Level Inverter/1
  connections:
  2 Level Inverter/RConn1 -- +/RConn1
  2 Level Inverter/RConn2 -- -/RConn1
  Series RLC Branch2/LConn1 -- 2 Level Inverter/LConn1
  2 Level Inverter/LConn2 -- Series RLC Branch1/LConn1
  2 Level Inverter/LConn3 -- Series RLC Branch3/LConn1
  Series RLC Branch2/RConn1 -- AC Load Measurements/LConn1
  Series RLC Branch1/RConn1 -- AC Load Measurements/LConn2
  Series RLC Branch3/RConn1 -- AC Load Measurements/LConn3
  AC Load Measurements/RConn1 -- A/RConn1
  AC Load Measurements/RConn2 -- B/RConn1
  AC Load Measurements/RConn3 -- C/RConn1

== system Microgrid_24h_Simulation/Inverter/DC BUS  ==
  Current Measurement1 : powerlib/Measurements/Current Measurement  PhasorSimulation=off  OutputType=Complex  PSBequivalent=0
      settings: SourceProductName=Simscape Electrical
  DC Bus : powerlib/Elements/Series RLC Branch  LConnTagsString=__new0  RConnTagsString=__new0  BranchType=C  Resistance=1  Inductance=5e-03  SetiL0=off  InitialCurrent=0  Capacitance=10e-3/2  Setx0=off  InitialVoltage=1000/2  Measurements=None
      settings: SourceProductName=Simscape Electrical
  "DC Bus " : powerlib/Elements/Series RLC Branch  LConnTagsString=__new0  RConnTagsString=__new0  BranchType=C  Resistance=1  Inductance=5e-03  SetiL0=off  InitialCurrent=0  Capacitance=10e-3/2  Setx0=off  InitialVoltage=1000/2  Measurements=None
      settings: SourceProductName=Simscape Electrical
  Ground : powerlib/Elements/Ground  LConnTagsString=a
      settings: SourceProductName=Simscape Electrical
  Subsystem1 : Subsystem
  Subsystem2 : Subsystem
  Voltage Measurement1 : powerlib/Measurements/Voltage Measurement  PhasorSimulation=off  OutputType=Complex  PSBequivalent=0
      settings: SourceProductName=Simscape Electrical
  "+ " : PMIOPort  Side=Left
  "- " : PMIOPort  Port=2  Side=Left
  "+  " : PMIOPort  Port=3  Side=Right
  "-  " : PMIOPort  Port=4  Side=Right
  wires:
  Voltage Measurement1/1 -> Subsystem2/1(Vdcinv)
  Current Measurement1/1 -> Subsystem1/1(Idcinv)
  connections:
  DC Bus/LConn1 -- "+  "/RConn1 -- Voltage Measurement1/LConn1 -- Current Measurement1/LConn1
  "DC Bus "/LConn1 -- DC Bus/RConn1 -- Ground/LConn1
  "DC Bus "/RConn1 -- "-  "/RConn1 -- "- "/RConn1 -- Voltage Measurement1/LConn2
  Current Measurement1/RConn1 -- "+ "/RConn1

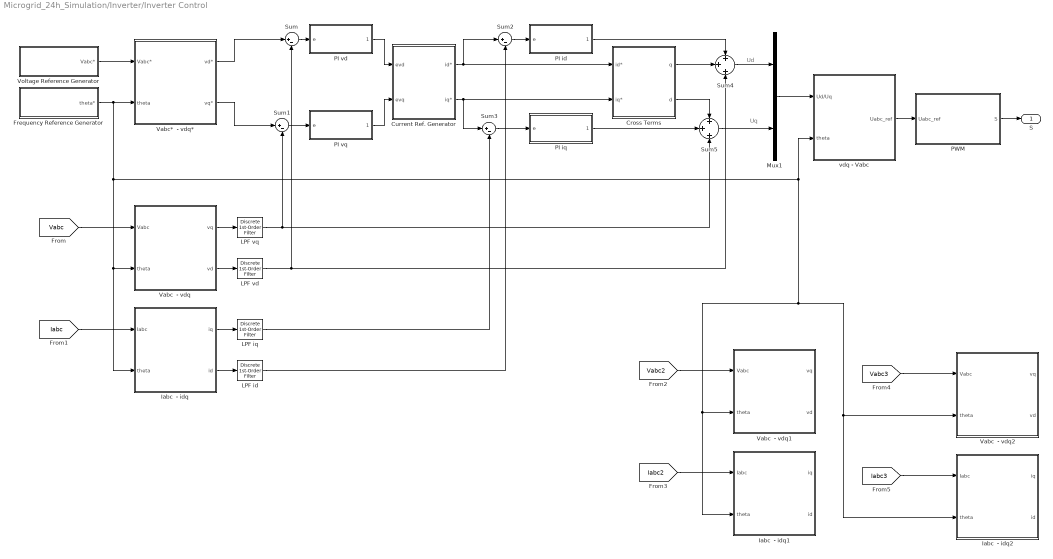
== system Microgrid_24h_Simulation/Inverter/Inverter Control ==
  note: Ud
  note: Uq
  " Voltage Reference Generator" : Subsystem
  Cross Terms : Subsystem
  Current Ref. Generator : Subsystem
  Frequency Reference Generator : Subsystem
  Iabc  - idq : Subsystem
  Iabc  - idq1 : Subsystem
  Iabc  - idq2 : Subsystem
  LPF id : powerlib_extras/Discrete  Control Blocks/Discrete 1st-Order Filter  FilterType=Lowpass  Tc=1e-3  Ts=5e-6  Initialize=off  Vac_Init=[0.8 -25 60]  Vdc_Init=0  PlotResponse=off  param1=[1 100 0.1]
      settings: SourceProductName=Simscape Electrical  SourceProductBaseCode=PS
  LPF iq : powerlib_extras/Discrete  Control Blocks/Discrete 1st-Order Filter  FilterType=Lowpass  Tc=1e-3  Ts=5e-6  Initialize=off  Vac_Init=[0.8 -25 60]  Vdc_Init=0  PlotResponse=off  param1=[1 100 0.1]
      settings: SourceProductName=Simscape Electrical  SourceProductBaseCode=PS
  LPF vd : powerlib_extras/Discrete  Control Blocks/Discrete 1st-Order Filter  FilterType=Lowpass  Tc=10e-3  Ts=5e-6  Initialize=off  Vac_Init=[0.8 -25 60]  Vdc_Init=-0.4  PlotResponse=off  param1=[1 100 0.1]
      settings: SourceProductName=Simscape Electrical  SourceProductBaseCode=PS
  LPF vq : powerlib_extras/Discrete  Control Blocks/Discrete 1st-Order Filter  FilterType=Lowpass  Tc=10e-3  Ts=5e-6  Initialize=off  Vac_Init=[0.8 -25 60]  Vdc_Init=0  PlotResponse=off  param1=[1 100 0.1]
      settings: SourceProductName=Simscape Electrical  SourceProductBaseCode=PS
  Mux1 : Mux  Inputs=2
  PI id : Subsystem
  PI iq : Subsystem
  PI vd : Subsystem
  PI vq : Subsystem
  PWM : Subsystem
  Sum{,1..3} (4 alike) : Sum  Inputs=|+-
  Sum4 : Sum  Inputs=+|+|+
  Sum5 : Sum  Inputs=+|+|+
  Vabc  - vdq : Subsystem
  Vabc  - vdq1 : Subsystem
  Vabc  - vdq2 : Subsystem
  Vabc*  - vdq* : Subsystem
  vdq - Vabc : Subsystem
  S : Outport
  wires:
  [Vabc] -> Vabc  - vdq/1(Vabc)
  [Iabc] -> Iabc  - idq/1(Iabc)
  Sum2/1 -> PI id/1(e)
  Sum3/1 -> PI iq/1(e)
  Mux1/1 -> vdq - Vabc/1(Ud/Uq)
  vdq - Vabc/1(Uabc_ref) -> PWM/1(Uabc_ref)
  PWM/1(S) -> S/1
  Vabc  - vdq/2(vd) -> LPF vd/1
  Iabc  - idq/1(iq) -> LPF iq/1
  Iabc  - idq/2(id) -> LPF id/1
  LPF vd/1 -> Sum/2, Sum4/3
  LPF vq/1 -> Sum1/2, Sum5/3
  LPF iq/1 -> Sum3/2
  LPF id/1 -> Sum2/2
  Sum/1 -> PI vd/1(e)
  Sum1/1 -> PI vq/1(e)
  Vabc  - vdq/1(vq) -> LPF vq/1
  Vabc*  - vdq*/1(vd*) -> Sum/1
  Vabc*  - vdq*/2(vq*) -> Sum1/1
  " Voltage Reference Generator"/1(Vabc*) -> Vabc*  - vdq*/1(Vabc*)
  Frequency Reference Generator/1(theta*) -> Vabc*  - vdq*/2(theta), Vabc  - vdq/2(theta), Iabc  - idq/2(theta), vdq - Vabc/2(theta), Vabc  - vdq2/2(theta), Iabc  - idq2/2(theta), Iabc  - idq1/2(theta), Vabc  - vdq1/2(theta)
  PI vd/1(" ") -> Current Ref. Generator/1(evd)
  PI vq/1(" ") -> Current Ref. Generator/2(evq)
  Current Ref. Generator/2(iq*) -> Sum3/1, Cross Terms/2(iq*)
  Current Ref. Generator/1(id*) -> Sum2/1, Cross Terms/1(id*)
  PI iq/1(" ") -> Sum5/2
  PI id/1(" ") -> Sum4/1
  Cross Terms/1(" q") -> Sum4/2
  Cross Terms/2(" d") -> Sum5/1
  Sum5/1 -> Mux1/2
  Sum4/1 -> Mux1/1
  [Vabc2] -> Vabc  - vdq1/1(Vabc)
  [Iabc2] -> Iabc  - idq1/1(Iabc)
  [Vabc3] -> Vabc  - vdq2/1(Vabc)
  [Iabc3] -> Iabc  - idq2/1(Iabc)

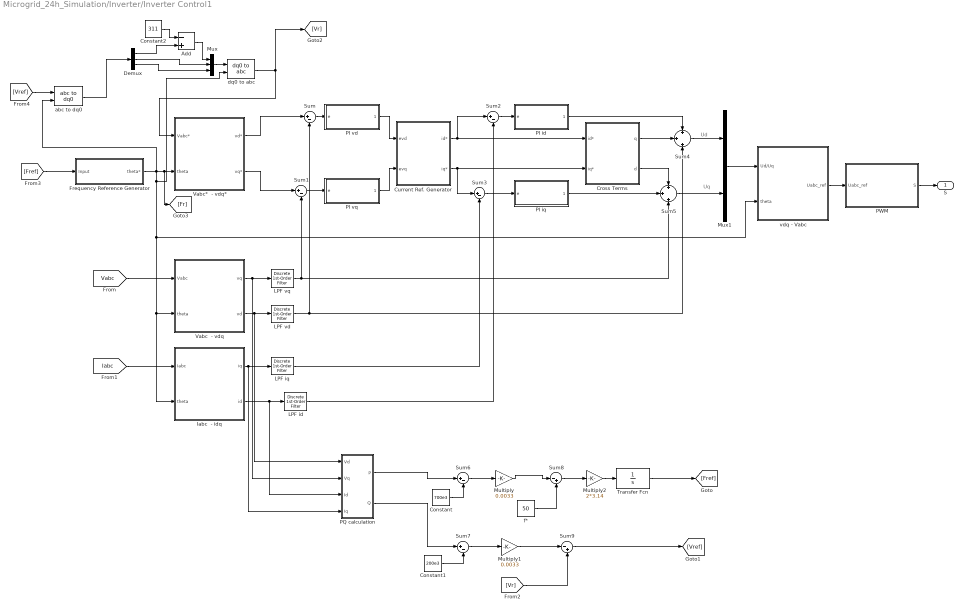
== system Microgrid_24h_Simulation/Inverter/Inverter Control1 ==
  note: Ud
  note: Uq
  Add : Sum  Inputs=-+
  Constant : Constant  Value=700e3
  Constant1 : Constant  Value=200e3
  Constant2 : Constant  Value=311
  Cross Terms : Subsystem
  Current Ref. Generator : Subsystem
  Demux : Demux  Outputs=3
  Frequency Reference Generator : Subsystem
  Iabc  - idq : Subsystem
  LPF id : powerlib_extras/Discrete  Control Blocks/Discrete 1st-Order Filter  FilterType=Lowpass  Tc=1e-3  Ts=5e-6  Initialize=off  Vac_Init=[0.8 -25 60]  Vdc_Init=0  PlotResponse=off  param1=[1 100 0.1]
      settings: SourceProductName=Simscape Electrical  SourceProductBaseCode=PS
  LPF iq : powerlib_extras/Discrete  Control Blocks/Discrete 1st-Order Filter  FilterType=Lowpass  Tc=1e-3  Ts=5e-6  Initialize=off  Vac_Init=[0.8 -25 60]  Vdc_Init=0  PlotResponse=off  param1=[1 100 0.1]
      settings: SourceProductName=Simscape Electrical  SourceProductBaseCode=PS
  LPF vd : powerlib_extras/Discrete  Control Blocks/Discrete 1st-Order Filter  FilterType=Lowpass  Tc=10e-3  Ts=5e-6  Initialize=off  Vac_Init=[0.8 -25 60]  Vdc_Init=-0.4  PlotResponse=off  param1=[1 100 0.1]
      settings: SourceProductName=Simscape Electrical  SourceProductBaseCode=PS
  LPF vq : powerlib_extras/Discrete  Control Blocks/Discrete 1st-Order Filter  FilterType=Lowpass  Tc=10e-3  Ts=5e-6  Initialize=off  Vac_Init=[0.8 -25 60]  Vdc_Init=0  PlotResponse=off  param1=[1 100 0.1]
      settings: SourceProductName=Simscape Electrical  SourceProductBaseCode=PS
  Multiply : Gain  Gain=0.0033
  Multiply1 : Gain  Gain=0.0033
  Multiply2 : Gain  Gain=2*3.14
  Mux : Mux  Inputs=3
  Mux1 : Mux  Inputs=2
  PI id : Subsystem
  PI iq : Subsystem
  PI vd : Subsystem
  PI vq : Subsystem
  PQ calculation : Subsystem
  PWM : Subsystem
  Sum{,1..3,6..7} (6 alike) : Sum  Inputs=|+-
  Sum4 : Sum  Inputs=+|+|+
  Sum5 : Sum  Inputs=+|+|+
  Sum8 : Sum  Inputs=|-+
  Sum9 : Sum  Inputs=|-+
  Transfer Fcn : TransferFcn  Denominator=[0 1 0]
  Vabc  - vdq : Subsystem
  Vabc*  - vdq* : Subsystem
  abc to dq0 : powerlib_meascontrol/Transformations/abc to dq0  Alignment=90 degrees behind phase A axis
      settings: SourceProductName=Simscape Electrical
  dq0 to abc : powerlib_meascontrol/Transformations/dq0 to abc  Alignment=90 degrees behind phase A axis
      settings: SourceProductName=Simscape Electrical
  "f* " : Constant  Value=50
  vdq - Vabc : Subsystem
  S : Outport
  wires:
  [Vabc] -> Vabc  - vdq/1(Vabc)
  [Iabc] -> Iabc  - idq/1(Iabc)
  Sum2/1 -> PI id/1(e)
  Sum3/1 -> PI iq/1(e)
  Mux1/1 -> vdq - Vabc/1(Ud/Uq)
  vdq - Vabc/1(Uabc_ref) -> PWM/1(Uabc_ref)
  PWM/1(S) -> S/1
  Vabc  - vdq/2(vd) -> PQ calculation/1(Vd), LPF vd/1
  Iabc  - idq/1(iq) -> PQ calculation/4(Iq), LPF iq/1
  Iabc  - idq/2(id) -> PQ calculation/3(Id), LPF id/1
  LPF vd/1 -> Sum/2, Sum4/3
  LPF vq/1 -> Sum1/2, Sum5/3
  LPF iq/1 -> Sum3/2
  LPF id/1 -> Sum2/2
  Sum/1 -> PI vd/1(e)
  Sum1/1 -> PI vq/1(e)
  Vabc  - vdq/1(vq) -> PQ calculation/2(Vq), LPF vq/1
  Vabc*  - vdq*/1(vd*) -> Sum/1
  Vabc*  - vdq*/2(vq*) -> Sum1/1
  dq0 to abc/1 -> [Vr], Vabc*  - vdq*/1(Vabc*)
  Frequency Reference Generator/1(theta*) -> dq0 to abc/2, Vabc  - vdq/2(theta), Iabc  - idq/2(theta), vdq - Vabc/2(theta), abc to dq0/2, [Fr], Vabc*  - vdq*/2(theta)
  PI vd/1(" ") -> Current Ref. Generator/1(evd)
  PI vq/1(" ") -> Current Ref. Generator/2(evq)
  Current Ref. Generator/2(iq*) -> Sum3/1, Cross Terms/2(iq*)
  Current Ref. Generator/1(id*) -> Sum2/1, Cross Terms/1(id*)
  PI iq/1(" ") -> Sum5/2
  PI id/1(" ") -> Sum4/1
  Cross Terms/1(" q") -> Sum4/2
  Cross Terms/2(" d") -> Sum5/1
  Sum5/1 -> Mux1/2
  Sum4/1 -> Mux1/1
  Constant1/1 -> Sum7/2
  Sum8/1 -> Multiply2/1
  Multiply/1 -> Sum8/1
  Multiply2/1 -> Transfer Fcn/1
  Constant/1 -> Sum6/2
  [Vr] -> Sum9/2
  "f* "/1 -> Sum8/2
  Sum7/1 -> Multiply1/1
  Multiply1/1 -> Sum9/1
  Sum6/1 -> Multiply/1
  PQ calculation/1(P) -> Sum6/1
  PQ calculation/2(Q) -> Sum7/1
  Transfer Fcn/1 -> [Fref]
  Sum9/1 -> [Vref]
  [Fref] -> Frequency Reference Generator/1(Input)
  [Vref] -> abc to dq0/1
  abc to dq0/1 -> Demux/1
  Constant2/1 -> Add/1
  Demux/1 -> Add/2
  Add/1 -> Mux/1
  Demux/2 -> Mux/2
  Demux/3 -> Mux/3
  Mux/1 -> dq0 to abc/1

== system Microgrid_24h_Simulation/PV Array/Subsystem1 ==
  Vpv : Inport
  LPF vq2 : powerlib_extras/Discrete  Control Blocks/Discrete 1st-Order Filter  FilterType=Lowpass  Tc=10e-3  Ts=5e-6  Initialize=off  Vac_Init=[0.8 -25 60]  Vdc_Init=0  PlotResponse=off  param1=[1 100 0.1]
      settings: SourceProductName=Simscape Electrical  SourceProductBaseCode=PS
  To Workspace1 : ToWorkspace  VariableName=Vpv  SampleTime=-1
  tag scope: Vpv=global
  wires:
  Vpv/1 -> [Vpv], LPF vq2/1
  LPF vq2/1 -> To Workspace1/1

== system Microgrid_24h_Simulation/PV Array/Subsystem2 ==
  Irr : Inport
  To Workspace1 : ToWorkspace  VariableName=Irr  SampleTime=-1
  Zero-Order Hold : ZeroOrderHold  SampleTime=5e-6
  tag scope: Irr=global
  wires:
  Irr/1 -> Zero-Order Hold/1
  Zero-Order Hold/1 -> To Workspace1/1, [Irr]

== system Microgrid_24h_Simulation/PV Array/Subsystem4 ==
  Ipv : Inport
  To Workspace1 : ToWorkspace  VariableName=Ipv_array  SampleTime=-1
  tag scope: Ipv_array=global
  wires:
  Ipv/1 -> [Ipv_array], To Workspace1/1

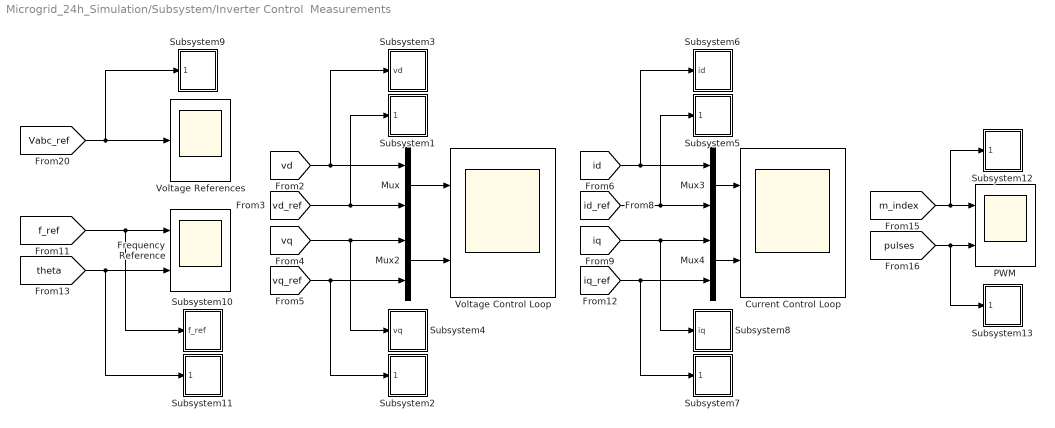
== system Microgrid_24h_Simulation/Subsystem/Inverter Control  Measurements ==
  Current Control Loop : Scope  NumInputPorts=2
  Frequency Reference : Scope  NumInputPorts=2
  Mux{,2..4} (4 alike) : Mux  Inputs=2
  PWM : Scope  NumInputPorts=2
  Subsystem1 : Subsystem
  Subsystem10 : Subsystem
  Subsystem11 : Subsystem
  Subsystem12 : Subsystem
  Subsystem13 : Subsystem
  Subsystem2 : Subsystem
  Subsystem3 : Subsystem
  Subsystem4 : Subsystem
  Subsystem5 : Subsystem
  Subsystem6 : Subsystem
  Subsystem7 : Subsystem
  Subsystem8 : Subsystem
  Subsystem9 : Subsystem
  Voltage Control Loop : Scope  NumInputPorts=2
  Voltage References : Scope
  wires:
  [vd] -> Mux/1, Subsystem3/1(vd)
  [vd_ref] -> Mux/2, Subsystem1/1(vd_ref)
  [vq] -> Mux2/1, Subsystem4/1(vq)
  [vq_ref] -> Mux2/2, Subsystem2/1(vq_ref)
  Mux/1 -> Voltage Control Loop/1
  Mux2/1 -> Voltage Control Loop/2
  [id] -> Mux3/1, Subsystem6/1(id)
  [id_ref] -> Mux3/2, Subsystem5/1(id_ref)
  [iq] -> Mux4/1, Subsystem8/1(iq)
  [iq_ref] -> Mux4/2, Subsystem7/1(iq_ref)
  [Vabc_ref] -> Voltage References/1, Subsystem9/1(Vabc_ref)
  Mux3/1 -> Current Control Loop/1
  Mux4/1 -> Current Control Loop/2
  [theta] -> Frequency Reference/2, Subsystem11/1(theta)
  [f_ref] -> Frequency Reference/1, Subsystem10/1(f_ref)
  [pulses] -> PWM/2, Subsystem13/1(pulses)
  [m_index] -> PWM/1, Subsystem12/1(m_index)

== system Microgrid_24h_Simulation/Subsystem/Inverter Control  Measurements1 ==
  Boost Converter Control MPPT : Scope  NumInputPorts=3
  wires:
  [Vref] -> Boost Converter Control MPPT/1
  [delta] -> Boost Converter Control MPPT/2
  [pulsos] -> Boost Converter Control MPPT/3

== system Microgrid_24h_Simulation/Subsystem/Inverter Control  Measurements2 ==
  Control Loops : Scope  NumInputPorts=2
  Mux : Mux  Inputs=2
  Mux2 : Mux  Inputs=2
  Switch Control : Scope  NumInputPorts=3
  wires:
  [Vdc] -> Mux/1
  [Vdc_ref] -> Mux/2
  [Ibat] -> Mux2/1
  [Ibat_ref] -> Mux2/2
  Mux/1 -> Control Loops/1
  Mux2/1 -> Control Loops/2
  [Sign] -> Switch Control/1
  [S1] -> Switch Control/2
  [S2] -> Switch Control/3

== system Microgrid_24h_Simulation/Subsystem/Inverter Control  Measurements3 ==
  PLL : Subsystem
  Subsystem : Subsystem
  wires:
  Subsystem/1(Vabc) -> PLL/1(Vabc)

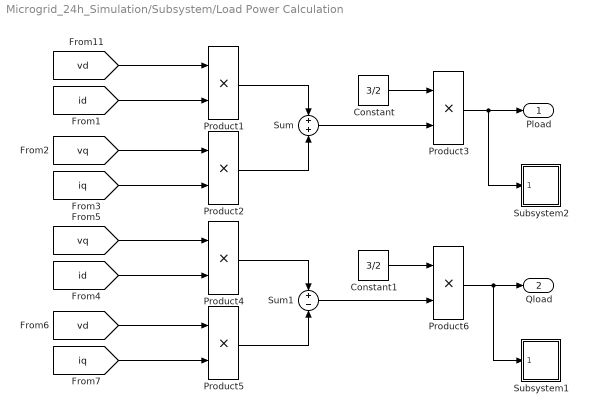
== system Microgrid_24h_Simulation/Subsystem/Load Power Calculation ==
  Constant : Constant  Value=3/2
  Constant1 : Constant  Value=3/2
  Product{1..6} (6 alike) : Product  RndMeth=Zero
  Subsystem1 : Subsystem
  Subsystem2 : Subsystem
  Sum : Sum  Inputs=+|+
  Sum1 : Sum  Inputs=+|-
  Pload : Outport
  Qload : Outport  Port=2
  wires:
  [vd] -> Product1/1
  [id] -> Product1/2
  [vq] -> Product2/1
  [iq] -> Product2/2
  Product1/1 -> Sum/1
  Product2/1 -> Sum/2
  Sum/1 -> Product3/2
  Constant/1 -> Product3/1
  Product3/1 -> Pload/1, Subsystem2/1(Pload)
  [vq] -> Product4/1
  [id] -> Product4/2
  [vd] -> Product5/1
  [iq] -> Product5/2
  Product4/1 -> Sum1/1
  Product5/1 -> Sum1/2
  Sum1/1 -> Product6/2
  Constant1/1 -> Product6/1
  Product6/1 -> Qload/1, Subsystem1/1(Qacload)

== system Microgrid_24h_Simulation/Subsystem/Subsystem ==
  Mux : Mux  Inputs=3
  Vabc : Outport
  wires:
  Mux/1 -> Vabc/1
  [Vab] -> Mux/1
  [Vbc] -> Mux/2
  [Vca] -> Mux/3

== system Microgrid_24h_Simulation/Subsystem/Subsystem1 ==
  Pbus : Inport
  LPF vq11 : powerlib_extras/Discrete  Control Blocks/Discrete 1st-Order Filter  FilterType=Lowpass  Tc=10e-3  Ts=5e-6  Initialize=off  Vac_Init=[0.8 -25 60]  Vdc_Init=0  PlotResponse=off  param1=[1 100 0.1]
      settings: SourceProductName=Simscape Electrical  SourceProductBaseCode=PS
  To Workspace1 : ToWorkspace  VariableName=Pbus  SampleTime=-1
  To Workspace2 : ToWorkspace  VariableName=Pbus1  SampleTime=-1
  tag scope: Pbus=global
  wires:
  Pbus/1 -> [Pbus], To Workspace1/1, LPF vq11/1
  LPF vq11/1 -> To Workspace2/1

== system Microgrid_24h_Simulation/Subsystem/Subsystem10 ==
  f : Inport
  LPF vq7 : powerlib_extras/Discrete  Control Blocks/Discrete 1st-Order Filter  FilterType=Lowpass  Tc=10e-3  Ts=5e-6  Initialize=off  Vac_Init=[0.8 -25 60]  Vdc_Init=0  PlotResponse=off  param1=[1 100 0.1]
      settings: SourceProductName=Simscape Electrical  SourceProductBaseCode=PS
  To Workspace1 : ToWorkspace  VariableName=fabc_real  SampleTime=-1
  To Workspace2 : ToWorkspace  VariableName=fabc_real_fil  SampleTime=-1
  Zero-Order Hold : ZeroOrderHold  SampleTime=5e-6
  wires:
  f/1 -> Zero-Order Hold/1
  LPF vq7/1 -> To Workspace2/1
  Zero-Order Hold/1 -> To Workspace1/1, LPF vq7/1

== system Microgrid_24h_Simulation/Subsystem/Subsystem11 ==
  LPF vq{2..3,8..9} (4 alike) : powerlib_extras/Discrete  Control Blocks/Discrete 1st-Order Filter  FilterType=Lowpass  Tc=10e-3  Ts=5e-6  Initialize=off  Vac_Init=[0.8 -25 60]  Vdc_Init=0  PlotResponse=off  param1=[1 100 0.1]
      settings: SourceProductName=Simscape Electrical  SourceProductBaseCode=PS
  Load Measurements1 : Scope  NumInputPorts=2
  Load Measurements3 : Scope  NumInputPorts=2
  Load Power Calculation1 : Subsystem
  Load Power Calculation2 : Subsystem
  Load Powers1 : Scope  NumInputPorts=2
  Load Powers2 : Scope  NumInputPorts=2
  wires:
  [Vabc2] -> Load Measurements1/1
  [Iabc2] -> Load Measurements1/2
  Load Power Calculation1/1(Pload) -> LPF vq2/1
  Load Power Calculation1/2(Qload) -> LPF vq3/1
  LPF vq2/1 -> Load Powers1/1
  LPF vq3/1 -> Load Powers1/2
  [Vabc3] -> Load Measurements3/1
  [Iabc3] -> Load Measurements3/2
  Load Power Calculation2/1(Pload) -> LPF vq8/1
  Load Power Calculation2/2(Qload) -> LPF vq9/1
  LPF vq8/1 -> Load Powers2/1
  LPF vq9/1 -> Load Powers2/2

== system Microgrid_24h_Simulation/Subsystem/Subsystem3 ==
  Pdc : Inport
  LPF vq7 : powerlib_extras/Discrete  Control Blocks/Discrete 1st-Order Filter  FilterType=Lowpass  Tc=10e-3  Ts=5e-6  Initialize=off  Vac_Init=[0.8 -25 60]  Vdc_Init=0  PlotResponse=off  param1=[1 100 0.1]
      settings: SourceProductName=Simscape Electrical  SourceProductBaseCode=PS
  To Workspace1 : ToWorkspace  VariableName=Pdc  SampleTime=-1
  To Workspace2 : ToWorkspace  VariableName=Pdc1  SampleTime=-1
  tag scope: Pdc=global
  wires:
  Pdc/1 -> [Pdc], To Workspace1/1, LPF vq7/1
  LPF vq7/1 -> To Workspace2/1

== system Microgrid_24h_Simulation/Subsystem/Subsystem4 ==
  Ppv : Inport
  LPF vq7 : powerlib_extras/Discrete  Control Blocks/Discrete 1st-Order Filter  FilterType=Lowpass  Tc=10e-3  Ts=5e-6  Initialize=off  Vac_Init=[0.8 -25 60]  Vdc_Init=0  PlotResponse=off  param1=[1 100 0.1]
      settings: SourceProductName=Simscape Electrical  SourceProductBaseCode=PS
  To Workspace1 : ToWorkspace  VariableName=Ppv  SampleTime=-1
  To Workspace2 : ToWorkspace  VariableName=Ppv1  SampleTime=-1
  tag scope: Ppv=global
  wires:
  Ppv/1 -> [Ppv], To Workspace1/1, LPF vq7/1
  LPF vq7/1 -> To Workspace2/1

== system Microgrid_24h_Simulation/Subsystem/Subsystem5 ==
  Pbat : Inport
  LPF vq7 : powerlib_extras/Discrete  Control Blocks/Discrete 1st-Order Filter  FilterType=Lowpass  Tc=10e-3  Ts=5e-6  Initialize=off  Vac_Init=[0.8 -25 60]  Vdc_Init=0  PlotResponse=off  param1=[1 100 0.1]
      settings: SourceProductName=Simscape Electrical  SourceProductBaseCode=PS
  To Workspace1 : ToWorkspace  VariableName=Pbat  SampleTime=-1
  To Workspace2 : ToWorkspace  VariableName=Pbat1  SampleTime=-1
  tag scope: Pbat=global
  wires:
  Pbat/1 -> [Pbat], To Workspace1/1, LPF vq7/1
  LPF vq7/1 -> To Workspace2/1

== system Microgrid_24h_Simulation/Subsystem/Subsystem6 ==
  Vab_rms : Inport
  To Workspace1 : ToWorkspace  VariableName=Vab_rms  SampleTime=-1
  tag scope: Vab_rms=global
  wires:
  Vab_rms/1 -> To Workspace1/1, [Vab_rms]

== system Microgrid_24h_Simulation/Subsystem/Subsystem7 ==
  Va_rms : Inport
  To Workspace1 : ToWorkspace  VariableName=Va_rms  SampleTime=-1
  tag scope: Va_rms=global
  wires:
  Va_rms/1 -> [Va_rms], To Workspace1/1

== system Microgrid_24h_Simulation/Subsystem/Subsystem8 ==
  Pdcinv : Inport
  LPF vq7 : powerlib_extras/Discrete  Control Blocks/Discrete 1st-Order Filter  FilterType=Lowpass  Tc=10e-3  Ts=5e-6  Initialize=off  Vac_Init=[0.8 -25 60]  Vdc_Init=0  PlotResponse=off  param1=[1 100 0.1]
      settings: SourceProductName=Simscape Electrical  SourceProductBaseCode=PS
  To Workspace1 : ToWorkspace  VariableName=Pdcinv  SampleTime=-1
  To Workspace2 : ToWorkspace  VariableName=Pdcinv1  SampleTime=-1
  tag scope: Pdcinv=global
  wires:
  Pdcinv/1 -> [Pdcinv], To Workspace1/1, LPF vq7/1
  LPF vq7/1 -> To Workspace2/1

== system Microgrid_24h_Simulation/Subsystem/Subsystem9 ==
  Mux1 : Mux  Inputs=3
  Iabc : Outport
  wires:
  [Ia] -> Mux1/1
  [Ib] -> Mux1/2
  [Ic] -> Mux1/3
  Mux1/1 -> Iabc/1

== system Microgrid_24h_Simulation/AC Load/Load Measurements/Subsystem1 ==
  Vabc : Inport
  To Workspace1 : ToWorkspace  VariableName=Vabc2  SampleTime=-1
  tag scope: Vabc2=global
  wires:
  Vabc/1 -> To Workspace1/1, [Vabc2]
